simulink model "three_level_PWM_ac_dc_conv"  (R2019b)
settings: Solver=VariableStepAuto  StartTime=0.0  StopTime=0.05  RelTol=1e-3
libraries: powerlib x23, simulink x2, powerlib_extras x1
settings Model: SimulationMode=rapid-accelerator  Creator=SPS VISION  LastModifiedBy=SPS VISION
settings SolverCC: ZeroCrossAlgorithm=Adaptive
settings DebuggingCC: IgnoredZcDiagnostic=none

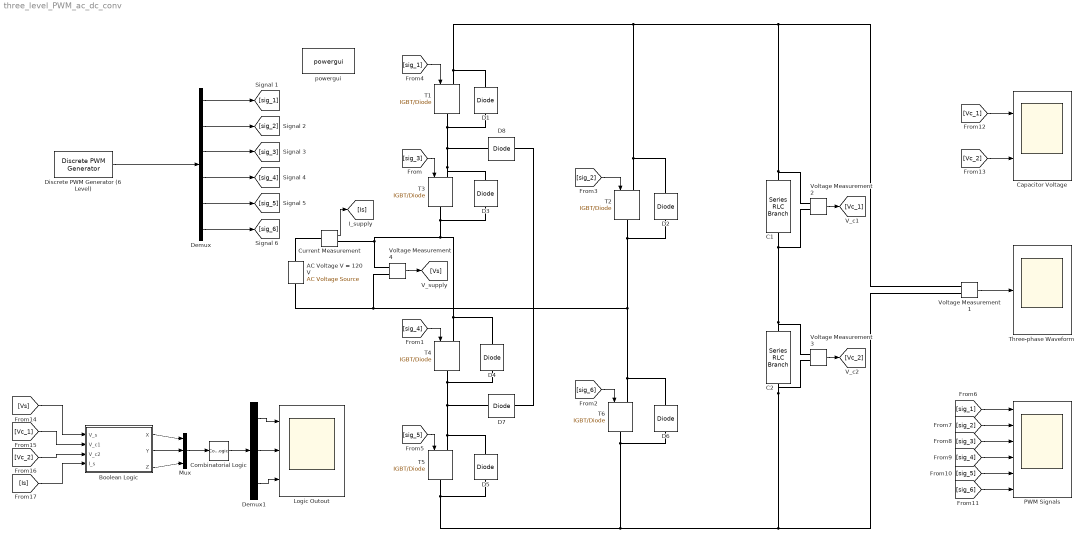
== system three_level_PWM_ac_dc_conv ==
  AC Voltage V = 120 V : powerlib/Electrical Sources/AC Voltage Source  Amplitude=120  Phase=0  Frequency=60  SampleTime=0  Measurements=None  BusType=swing  Pref=10e3  Qref=0  Qmin=-inf  Qmax=+inf
      settings: SourceProductName=Simscape Electrical
  Boolean Logic : Subsystem
  C1 : powerlib/Elements/Series RLC Branch  LConnTagsString=__new0  RConnTagsString=__new0  BranchType=C  Resistance=1  Inductance=5e-3  SetiL0=off  InitialCurrent=0  Capacitance=1e-6  Setx0=off  InitialVoltage=0  Measurements=Branch voltage
      settings: SourceProductName=Simscape Electrical
  C2 : powerlib/Elements/Series RLC Branch  LConnTagsString=__new0  RConnTagsString=__new0  BranchType=C  Resistance=1  Inductance=5e-3  SetiL0=off  InitialCurrent=0  Capacitance=1e-6  Setx0=off  InitialVoltage=0  Measurements=Branch voltage
      settings: SourceProductName=Simscape Electrical
  Capacitor Voltage : Scope  NumInputPorts=2
  Combinatorial Logic : CombinatorialLogic  TruthTable=[0 0 0; 0 0 1; 0 1 0; 0 1 1; 1 0 0; 1 0 1; 1 1 0; 1 1 1]
  Current Measurement : powerlib/Measurements/Current Measurement  PhasorSimulation=off  OutputType=Complex  PSBequivalent=0
      settings: SourceProductName=Simscape Electrical
  D{1..8} (8 alike) : powerlib/Power Electronics/Diode  Ron=0.001  Lon=0  Vf=0.8  IC=0  UseSnubber=off  Rs=500  Cs=250e-9  Measurements=off
      settings: SourceProductName=Simscape Electrical
  Demux : Demux  Outputs=6
  Demux1 : Demux  Outputs=3
  Discrete PWM Generator (6 Level) : powerlib_extras/Discrete  Control Blocks/Discrete PWM Generator  GeneratorMode="3-arm  bridge (6 pulses)"  Fc=600  Ts=5e-6  Internal=on  mIndex=0.5  Freq=60  Phase=0
      settings: SourceProductName=Simscape Electrical  SourceProductBaseCode=PS
  Logic Outout : Scope  NumInputPorts=3
  Mux : Mux  Inputs=3
  PWM Signals : Scope  NumInputPorts=6
  T{1..6} (6 alike) : powerlib/Power Electronics/IGBT//Diode  Ron=1e-3  Rs=1e5  Cs=inf  Measurements=off
      settings: SourceProductName=Simscape Electrical
  Three-phase Waveform : Scope
  Voltage Measurement{1..4} (4 alike) : powerlib/Measurements/Voltage Measurement  PhasorSimulation=off  OutputType=Complex  PSBequivalent=0
      settings: SourceProductName=Simscape Electrical
  powergui : powerlib/powergui  Priority=1  SimulationMode=Continuous  SampleTime=50e-6  frequency=60  Iterations=50  frequencyindice=0  Pbase=100e6  ErrMax=1e-4  UnitsV=kV  UnitsW=MW  buscounter=0  FunctionMessages=off  echomessages=off  EnableUseOfTLC=off  CurrentSourceSwitches=off  DisableSnubberDevices=off  DisableRonSwitches=off  DisableVfSwitches=off  DisplayEquations=off  AutomaticDiscreteSolvers=off  SolverType=Tustin/Backward Euler (TBE)  Interpol=off  ExternalGateDelay=off  methode=off  Ts=100  x0status=blocks  SPID=on  SwTol=0  HookPort=off  NonlinearTolerance=1e-4  nMaxIteration=100  ContinueOnMaxIteration=off  RestoreLinks=warning  ResistiveCurrentMeasurement=off  Frange=[0:2:500]  Ylog=off  Xlog=on  ShowGrid=off  save=off  variable=ZData  structure=Vout  ZoomFFT=off  StartTime=0.0  cycles=1  DisplayStyle=1  fundamental=60  FreqAxis=off  MaxFrequency=1000  frequencyindicesteady=1  RmsSteady=1  display=off
      settings: SourceProductName=Simscape Electrical
  wires:
  Demux/1 -> [sig_1]
  [sig_3] -> T3/1
  Demux/2 -> [sig_2]
  [sig_4] -> T4/1
  Voltage Measurement1/1 -> Three-phase Waveform/1
  [sig_6] -> T6/1
  [sig_2] -> T2/1
  Demux/3 -> [sig_3]
  [sig_1] -> T1/1
  [sig_5] -> T5/1
  Voltage Measurement2/1 -> [Vc_1]
  Voltage Measurement3/1 -> [Vc_2]
  Voltage Measurement4/1 -> [Vs]
  Current Measurement/1 -> [Is]
  Mux/1 -> Combinatorial Logic/1
  Boolean Logic/3(Z) -> Mux/3
  Boolean Logic/2(Y) -> Mux/2
  Boolean Logic/1(X) -> Mux/1
  Demux/4 -> [sig_4]
  Demux/5 -> [sig_5]
  Demux/6 -> [sig_6]
  [sig_1] -> PWM Signals/1
  [sig_2] -> PWM Signals/2
  [sig_3] -> PWM Signals/3
  [sig_4] -> PWM Signals/4
  [sig_5] -> PWM Signals/5
  [sig_6] -> PWM Signals/6
  [Vc_2] -> Capacitor Voltage/2
  [Vs] -> Boolean Logic/1(V_s)
  [Vc_1] -> Boolean Logic/2(V_c1)
  [Vc_2] -> Boolean Logic/3(V_c2)
  [Is] -> Boolean Logic/4(I_s)
  Discrete PWM Generator (6 Level)/1 -> Demux/1
  Combinatorial Logic/1 -> Demux1/1
  Demux1/1 -> Logic Outout/1
  Demux1/2 -> Logic Outout/2
  Demux1/3 -> Logic Outout/3
  [Vc_1] -> Capacitor Voltage/1
  connections:
  Current Measurement/RConn1 -- Voltage Measurement4/LConn1 -- D4/RConn1 -- T4/LConn1 -- D3/LConn1 -- T3/RConn1
  Voltage Measurement1/LConn2 -- Voltage Measurement3/LConn2 -- C2/RConn1 -- D5/LConn1 -- T5/RConn1 -- D6/LConn1 -- T6/RConn1
  D6/RConn1 -- T6/LConn1 -- D2/LConn1 -- T2/RConn1 -- Voltage Measurement4/LConn2 -- AC Voltage V = 120 V/LConn1
  T3/LConn1 -- D8/RConn1 -- D1/LConn1 -- T1/RConn1 -- D3/RConn1
  D4/LConn1 -- D7/LConn1 -- D5/RConn1 -- T5/LConn1 -- T4/RConn1
  T1/LConn1 -- D1/RConn1 -- Voltage Measurement2/LConn1 -- C1/LConn1 -- Voltage Measurement1/LConn1 -- D2/RConn1 -- T2/LConn1
  C1/RConn1 -- Voltage Measurement2/LConn2 -- Voltage Measurement3/LConn1 -- C2/LConn1
  D7/RConn1 -- D8/LConn1
  Current Measurement/LConn1 -- AC Voltage V = 120 V/RConn1

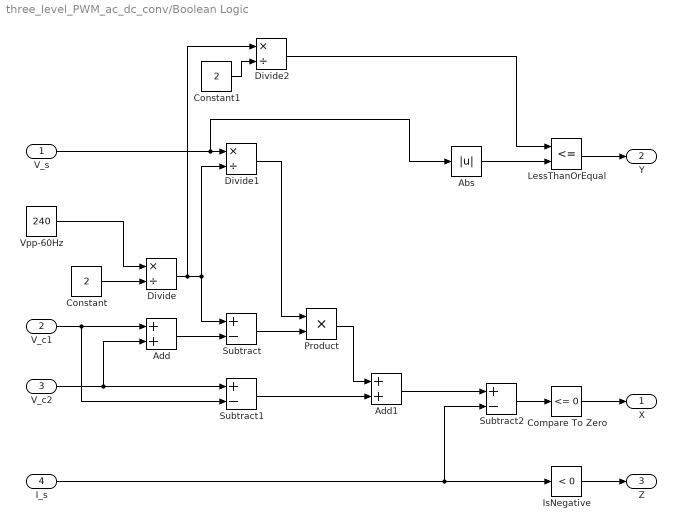
== system three_level_PWM_ac_dc_conv/Boolean Logic ==
  V_s : Inport
  V_c1 : Inport  Port=2
  V_c2 : Inport  Port=3
  I_s : Inport  Port=4
  Abs : Abs
  Add : Sum
  Add1 : Sum
  Compare To Zero : simulink/Logic and Bit Operations/Compare To Zero  relop=<=  OutDataTypeStr=boolean
  Constant : Constant  Value=2
  Constant1 : Constant  Value=2
  Divide : Product  Inputs=*/
  Divide1 : Product  Inputs=*/
  Divide2 : Product  Inputs=*/
  IsNegative : simulink/Logic and Bit Operations/Compare To Zero  relop=<  OutDataTypeStr=boolean
  LessThanOrEqual : RelationalOperator  Operator=<=  OutDataTypeStr=boolean  RndMeth=Simplest
  Product : Product
  Subtract : Sum  Inputs=+-
  Subtract1 : Sum  Inputs=+-
  Subtract2 : Sum  Inputs=+-
  Vpp-60Hz : Constant  Value=240
  X : Outport
  Y : Outport  Port=2
  Z : Outport  Port=3
  wires:
  Add/1 -> Subtract/2
  Constant/1 -> Divide/2
  Subtract1/1 -> Add1/2
  V_c1/1 -> Subtract1/2, Add/1
  V_c2/1 -> Subtract1/1, Add/2
  Vpp-60Hz/1 -> Divide/1
  Divide/1 -> Divide2/1, Divide1/2, Subtract/1
  Product/1 -> Add1/1
  Divide1/1 -> Product/1
  V_s/1 -> Abs/1, Divide1/1
  Subtract/1 -> Product/2
  Add1/1 -> Subtract2/1
  I_s/1 -> Subtract2/2, IsNegative/1
  Subtract2/1 -> Compare To Zero/1
  Abs/1 -> LessThanOrEqual/2
  Constant1/1 -> Divide2/2
  Divide2/1 -> LessThanOrEqual/1
  Compare To Zero/1 -> X/1
  LessThanOrEqual/1 -> Y/1
  IsNegative/1 -> Z/1
